simulink model "E33_VCU_simulink"  (R2014a)
settings: Solver=FixedStepDiscrete  StartTime=0.0  StopTime=10.0  FixedStep=0.0005  RelTol=1e-3
values from neighbouring files (symbols this model uses):
  Accu_FAN_Test = ecucoder_cal(Accu_FAN_Test)    [E33_VCU.m]
  Accu_FAN_threshold = ecucoder_cal(Accu_FAN_threshold)    [E33_VCU.m]
  APPS1_Voltage = ecucoder_cal(APPS1_Voltage)    [E33_VCU.m]
  APPS2_Voltage = ecucoder_cal(APPS2_Voltage)    [E33_VCU.m]
  APPS_Map = [0,1000]    [E33_VCU.m]
  APPS_threshold = ecucoder_cal(APPS_threshold)    [E33_VCU.m]
  Beep_Time = ecucoder_cal(Beep_Time)    [E33_VCU.m]
  BeeperTest = ecucoder_cal(BeeperTest)    [E33_VCU.m]
  BMSLedTest = ecucoder_cal(BMSLedTest)    [E33_VCU.m]
  BP_F_threshold = ecucoder_cal(BP_F_threshold)    [E33_VCU.m]
  BP_F_Voltage = ecucoder_cal(BP_F_Voltage)    [E33_VCU.m]
  BP_Map = [0,1000]    [E33_VCU.m]
  BP_R_Voltage = ecucoder_cal(BP_R_Voltage)    [E33_VCU.m]
  Brk_luminance = ecucoder_cal(Brk_luminance)    [E33_VCU.m]
  DCDC_Relay_Test = ecucoder_cal(DCDC_Relay_Test)    [E33_VCU.m]
  FactoryTestEnable = ecucoder_cal(FactoryTestEnable)    [E33_VCU.m]
  HardBrk_luminance = ecucoder_cal(HardBrk_luminance)    [E33_VCU.m]
  IMDLedTest = ecucoder_cal(IMDLedTest)    [E33_VCU.m]
  linear_FL_Map = ecucoder_cal(linear_FL_Map)    [E33_VCU.m]
  linear_FR_Map = ecucoder_cal(linear_FR_Map)    [E33_VCU.m]
  linear_Map = ecucoder_cal(linear_Map)    [E33_VCU.m]
  linear_RL_Map = ecucoder_cal(linear_RL_Map)    [E33_VCU.m]
  linear_RR_Map = ecucoder_cal(linear_RR_Map)    [E33_VCU.m]
  MaxPow = 40    [E33_VCU.m]
  MaxRPM = 5400    [E33_VCU.m]
  MaxRPMchangePerSec = ecucoder_cal(MaxRPMchangePerSec)    [E33_VCU.m]
  MaxTorqChangePerSec = ecucoder_cal(MaxTorqChangePerSec)    [E33_VCU.m]
  Motor_RPM_Map = (0:ceil(MaxRPM/100))*100    [E33_VCU.m]
  Pump_Test = ecucoder_cal(Pump_Test)    [E33_VCU.m]
  Pump_threshold = ecucoder_cal(Pump_threshold)    [E33_VCU.m]
  R2D_Light_Test = ecucoder_cal(R2D_Light_Test)    [E33_VCU.m]
  Radiator_FAN_Test = ecucoder_cal(Radiator_FAN_Test)    [E33_VCU.m]
  SCS_Error_5V = ecucoder_cal(SCS_Error_5V)    [E33_VCU.m]
  SCS_Error_GND = ecucoder_cal(SCS_Error_GND)    [E33_VCU.m]
  SPD_Coef = 1884/40    (= 47.1)    [E33_VCU.m]
  Tail_Light_Test = ecucoder_cal(Tail_Light_Test)    [E33_VCU.m]
  Tmanage_Map = [0,100]    [E33_VCU.m]
  Torq_percentage_Map = Motor_Torq_MAP/MaxTorq*1000    [E33_VCU.m]
libraries: simulink x164, ec55xxlib x44, dspswit3 x6
(part 5 of 5)

== system E33_VCU_simulink/Input/Input/MCU_CAN_Receive/ReceiveMessages/MCU_Stat/MCU_IsFreeMode_Sub ==
  In1 : Inport
  Out1 : Outport
  wires:
  In1/1 -> Out1/1

== system E33_VCU_simulink/Input/Input/MCU_CAN_Receive/ReceiveMessages/MCU_Stat/MCU_IsHvOvervoltage_Sub ==
  In1 : Inport
  Out1 : Outport
  wires:
  In1/1 -> Out1/1

== system E33_VCU_simulink/Input/Input/MCU_CAN_Receive/ReceiveMessages/MCU_Stat/MCU_IsHvUndervoltage_Sub ==
  In1 : Inport
  Out1 : Outport
  wires:
  In1/1 -> Out1/1

== system E33_VCU_simulink/Input/Input/MCU_CAN_Receive/ReceiveMessages/MCU_Stat/MCU_IsLvError_Sub ==
  In1 : Inport
  Out1 : Outport
  wires:
  In1/1 -> Out1/1

== system E33_VCU_simulink/Input/Input/MCU_CAN_Receive/ReceiveMessages/MCU_Stat/MCU_IsMcuNOTActive_Sub ==
  In1 : Inport
  Out1 : Outport
  wires:
  In1/1 -> Out1/1

== system E33_VCU_simulink/Input/Input/MCU_CAN_Receive/ReceiveMessages/MCU_Stat/MCU_IsMcuOvertemp_Sub ==
  In1 : Inport
  Out1 : Outport
  wires:
  In1/1 -> Out1/1

== system E33_VCU_simulink/Input/Input/MCU_CAN_Receive/ReceiveMessages/MCU_Stat/MCU_IsMotorOvertemp_Sub ==
  In1 : Inport
  Out1 : Outport
  wires:
  In1/1 -> Out1/1

== system E33_VCU_simulink/Input/Input/MCU_CAN_Receive/ReceiveMessages/MCU_Stat/MCU_IsOverCurr_Sub ==
  In1 : Inport
  Out1 : Outport
  wires:
  In1/1 -> Out1/1

== system E33_VCU_simulink/Input/Input/MCU_CAN_Receive/ReceiveMessages/MCU_Stat/MCU_IsPreChg_Sub ==
  In1 : Inport
  Out1 : Outport
  wires:
  In1/1 -> Out1/1

== system E33_VCU_simulink/Input/Input/MCU_CAN_Receive/ReceiveMessages/MCU_Stat/MCU_IsReady_Sub ==
  In1 : Inport
  Out1 : Outport
  wires:
  In1/1 -> Out1/1

== system E33_VCU_simulink/Input/Input/MCU_CAN_Receive/ReceiveMessages/MCU_Stat/MCU_IsRevoloverError_Sub ==
  In1 : Inport
  Out1 : Outport
  wires:
  In1/1 -> Out1/1

== system E33_VCU_simulink/Input/Input/MCU_CAN_Receive/ReceiveMessages/MCU_Stat/MCU_IsSelfcheckPass_Sub ==
  In1 : Inport
  Out1 : Outport
  wires:
  In1/1 -> Out1/1

== system E33_VCU_simulink/Input/Input/MCU_CAN_Receive/ReceiveMessages/MCU_Stat/MCU_IsSpdMode_Sub ==
  In1 : Inport
  Out1 : Outport
  wires:
  In1/1 -> Out1/1

== system E33_VCU_simulink/Input/Input/MCU_CAN_Receive/ReceiveMessages/MCU_Stat/MCU_IsTorqMode_Sub ==
  In1 : Inport
  Out1 : Outport
  wires:
  In1/1 -> Out1/1

== system E33_VCU_simulink/Input/Input/MCU_CAN_Receive/ReceiveMessages/MCU_Stat/MCU_IsUnderPowerLim_Sub ==
  In1 : Inport
  Out1 : Outport
  wires:
  In1/1 -> Out1/1

== system E33_VCU_simulink/Input/Input/MCU_CAN_Receive/ReceiveMessages/MCU_Stat/MCU_IsZeroLocMode_Sub ==
  In1 : Inport
  Out1 : Outport
  wires:
  In1/1 -> Out1/1

== system E33_VCU_simulink/Input/Input/MCU_CAN_Receive/ReceiveMessages/MCU_Stat/MCU_SPD_RPT_Sub ==
  In1 : Inport
  Out1 : Outport
  wires:
  In1/1 -> Out1/1

== system E33_VCU_simulink/Input/Input/MCU_CAN_Receive/ReceiveMessages/MCU_Stat/MCU_TORQ_RPT_Sub ==
  In1 : Inport
  Out1 : Outport
  wires:
  In1/1 -> Out1/1

== system E33_VCU_simulink/Input/Input/MCU_CAN_Receive/ReceiveMessages1/Enabled Subsystem/MCU_HvAcCurrRms_Sub ==
  In1 : Inport
  Out1 : Outport
  wires:
  In1/1 -> Out1/1

== system E33_VCU_simulink/Input/Input/MCU_CAN_Receive/ReceiveMessages1/Enabled Subsystem/MCU_HvCurr_Sub ==
  In1 : Inport
  Out1 : Outport
  wires:
  In1/1 -> Out1/1

== system E33_VCU_simulink/Input/Input/MCU_CAN_Receive/ReceiveMessages1/Enabled Subsystem/MCU_HvVolt_Sub ==
  In1 : Inport
  Out1 : Outport
  wires:
  In1/1 -> Out1/1

== system E33_VCU_simulink/Input/Input/MCU_CAN_Receive/ReceiveMessages1/Enabled Subsystem/MCU_McuTemp_Sub ==
  In1 : Inport
  Out1 : Outport
  wires:
  In1/1 -> Out1/1

== system E33_VCU_simulink/Input/Input/MCU_CAN_Receive/ReceiveMessages1/Enabled Subsystem/MCU_MotorTemp_Sub ==
  In1 : Inport
  Out1 : Outport
  wires:
  In1/1 -> Out1/1

== stateflow chart E33_VCU_simulink/Subsystem1/TmanageCtrl/Accu_FAN1 ==
  state LEDStat
    state Run
      du:FanDutyCycl = FanPwr
    state Init
    state PumpTest
      du:FanDutyCycl  = uint16(GetDutyCyc(temporalCount(sec),8));
    (default) -> Init
    Init -> PumpTest : after(1,sec)
    Run -> PumpTest : [IsPrechg]
    PumpTest -> Run : [after(2,sec)]
  data: elapsed_sec function_input; DutyCyc function_output uint8; period function_input; FanPwr input uint16; FanDutyCycl output uint16; IsPrechg input boolean; IsRun input
  function DutyCyc = GetDutyCyc(elapsed_sec, period):
    | function DutyCyc = GetDutyCyc(elapsed_sec, period)
    |     DutyCyc = 25.*sin(2.*pi.*(elapsed_sec./period+0.75))+25;      %Note: sin in rad
    | end

== stateflow chart E33_VCU_simulink/Function-Call Subsystem/R2D_State/Chart ==
  state VehStat [parallel]
    settings: executionOrder=1
    state Guard
    state Standby
    state WaitForEngine
    state Trans
    state Init
    state Ready
    Standby -> Guard [order 1] : [R2D_SW&&BP_F_OK&&APPS_OK]
    Guard -> Trans [order 1] : after(0.25,sec){send(EbeepON,BeeperStat)}
    WaitForEngine -> Standby : [MCU_Ready]
    Standby -> WaitForEngine [order 2] : [~MCU_Ready]
    Guard -> Standby [order 2] : [~R2D_SW||~BP_F_OK||~APPS_OK]
    Init -> WaitForEngine : [after(1,sec)]
    Ready -> WaitForEngine : [~MCU_Ready]
    Guard -> WaitForEngine [order 3] : [~MCU_Ready]
    Trans -> Ready : after(Beep_Time,sec){send(EbeepOFF,BeeperStat)}
    (default) -> Init
  state Output [parallel]
    du:
    VehStandby = in(VehStat.Standby);
    VehReady = in(VehStat.Ready);
    BeeperStOut = in(BeeperStat.ON);
    settings: executionOrder=3
  state BeeperStat [parallel]
    settings: executionOrder=2
    state OFF
    state ON
    (default) -> OFF
    OFF -> ON : EbeepON
    ON -> OFF : EbeepOFF
  data: BeeperStOut output boolean size=1; VehStandby output boolean; R2D_SW input boolean; APPS_OK input boolean; BP_F_OK input boolean; MCU_Ready input boolean; VehReady output boolean; Beep_Time input
  events: EbeepON local FUNCTION_CALL_EVENT; EbeepOFF local FUNCTION_CALL_EVENT

== stateflow chart E33_VCU_simulink/Subsystem1/TailLight/LED ==
  state LEDStat
    state Init
    state LightTest
      du:LEDDutyCyc  = uint16(GetDutyCyc(temporalCount(sec),4));
    state OFF
      entry: LEDDutyCyc = uint16(0);
    state Blink
      state BlinkOn
        entry: LEDDutyCyc = uint16(HardBrk_luminance);
      state BlinkOff
        entry: LEDDutyCyc = uint16(Brk_luminance);
      (default) -> BlinkOn
      BlinkOn -> BlinkOff : after(100,msec)
      BlinkOff -> BlinkOn : after(100,msec)
    state ON
      entry: LEDDutyCyc = uint16(Brk_luminance);
    (default) -> Init
    Init -> LightTest : after(1,sec)
    LightTest -> OFF : after(4,sec){LEDDutyCyc = uint16(0)}
    OFF -> Blink [order 1] : [IsHardBrk]
    Blink -> OFF [order 2] : [~IsBrk]
    OFF -> ON [order 2] : [IsBrk]
    ON -> OFF [order 1] : [~IsBrk]
    Blink -> ON [order 1] : [~IsHardBrk&&IsBrk]
    ON -> Blink [order 2] : [IsHardBrk]
  data: elapsed_sec function_input; DutyCyc function_output uint8; period function_input; IsBrk input boolean; LEDDutyCyc output uint16; IsHardBrk input boolean; Brk_luminance input double; HardBrk_luminance input double
  function DutyCyc = GetDutyCyc(elapsed_sec, period):
    | function DutyCyc = GetDutyCyc(elapsed_sec, period)
    |     DutyCyc = 25.*sin(2.*pi.*(elapsed_sec./period+0.75))+25;      %Note: sin in rad
    | end

== stateflow chart E33_VCU_simulink/Subsystem1/TmanageCtrl/Pump ==
  state Pump_MR
    state Init
    state OFF
      du:Pump_ON = 0
    state ON
      du:Pump_ON = 1
    state PumpTest
      du:Pump_ON  =  1
    (default) -> Init
    Init -> PumpTest : after(1,sec)
    OFF -> ON : [Pump_OK]
    PumpTest -> OFF : after(8,sec)
    ON -> OFF : [~Pump_OK]
  data: Pump_OK input boolean; MCU_IsReady input boolean; Pump_ON output

== stateflow chart E33_VCU_simulink/Subsystem1/PanelCtrl/Ready_SW ==
  state LEDStat
    state Blink
      state BlinkONslow
        entry: R2D_Light = true;
      state BlinkOFFslow
        entry: R2D_Light = false;
      (default) -> BlinkONslow
      BlinkONslow -> BlinkOFFslow : [after(1,sec)]
      BlinkOFFslow -> BlinkONslow : [after(1,sec)]
    state Init
      du: R2D_Light = false;
    state Test
      en:
      R2D_Light = true;
    state FastBlink
      state BlinkONfast
        entry: R2D_Light = true;
      state BlinkOFFfast
        entry: R2D_Light = false;
      (default) -> BlinkONfast
      BlinkONfast -> BlinkOFFfast : after(0.2,sec)
      BlinkOFFfast -> BlinkONfast : after(0.2,sec)
    state ON
      en:R2D_Light = true;
    state OFF
      en:R2D_Light = false;
    (junction 72) -> (junction 51)
    (junction 51) -> (junction 70)
    (junction 82) -> (junction 72)
    (default) -> Init
    Init -> Test : after(1,sec)
    Test -> (junction 70) : after(3,sec){R2D_Light = false}
    (junction 70) -> Blink [order 1] : [VehStandby]
    Blink -> (junction 82) : [APPS_Unreliable||~VehStandby]
    (junction 70) -> (junction 93) [order 2]
    (junction 96) -> (junction 82)
    (junction 93) -> FastBlink [order 1] : [APPS_Unreliable]
    FastBlink -> (junction 96) : [~APPS_Unreliable]
    (junction 78) -> (junction 96)
    (junction 93) -> (junction 73) [order 2]
    (junction 73) -> ON [order 1] : [VehReady]
    ON -> (junction 78)
    (junction 73) -> (junction 67) [order 2]
    (junction 59) -> (junction 78)
    (junction 67) -> OFF
    OFF -> (junction 59)
  data: R2D_Light output boolean; APPS_Unreliable input boolean; VehStandby input boolean; VehReady input boolean

== stateflow chart E33_VCU_simulink/Subsystem1/PanelCtrl/BMS_ALM ==
  state LEDStat
    state AlevelAlm
      en:LED = true;
    state Init
      en:
      LED = false;
    state BlevelAlm
      state BlvBlinkOff
        entry:
        LED = false;
      state BlvBlinkON
        entry:
        LED = true;
      BlvBlinkOff -> BlvBlinkON : after(1,sec)
      BlvBlinkON -> BlvBlinkOff : after(1,sec)
      (default) -> BlvBlinkON
    state Test
      en:
      LED = true;
    state OFF
      en:
      LED = false;
    (junction 55) -> (junction 56)
    (junction 56) -> (junction 15)
    (junction 47) -> (junction 55)
    (default) -> Init
    Test -> (junction 15) : after(3,sec){LED = true}
    (junction 15) -> AlevelAlm [order 1] : [AlmLv==1||~OK]
    (junction 15) -> (junction 32) [order 2]
    AlevelAlm -> (junction 47) : [AlmLv~=1&&OK]
    (junction 45) -> (junction 47)
    Init -> Test : after(1,sec)
    (junction 32) -> BlevelAlm [order 1] : [AlmLv==2]
    (junction 32) -> (junction 34) [order 2]
    BlevelAlm -> (junction 45) : [AlmLv~=2||~OK]
    (junction 41) -> (junction 45)
    (junction 34) -> OFF
    OFF -> (junction 41)
  data: AlmLv input; LED output boolean; OK input

== stateflow chart E33_VCU_simulink/Subsystem1/PanelCtrl/IMD_ALM ==
  state LEDStat
    state AlevelAlm
      en:LED = false;
    state Init
      en:
      LED = false;
    state OFF
      en:
      LED = true;
    state Test
      en:
      LED = true;
    (junction 55) -> (junction 56)
    (junction 56) -> (junction 15)
    (junction 47) -> (junction 55)
    (default) -> Init
    (junction 15) -> AlevelAlm [order 1] : [~OK]
    Test -> (junction 15) : after(3,sec){LED = true}
    (junction 15) -> (junction 34) [order 2]
    AlevelAlm -> (junction 47) : [OK]
    (junction 41) -> (junction 47)
    Init -> Test : after(1,sec)
    (junction 34) -> OFF
    OFF -> (junction 41)
  data: LED output boolean; OK input

== stateflow chart E33_VCU_simulink/Subsystem1/DCDC_Ctrl/DCDC_Ctrl ==
  state DCDC_MR
    du:DCDC_ON = in(DCDC_MR.ON)
    state OFF
    state ON
    (default) -> OFF
    OFF -> ON : [after(2,sec)&&HV_ON]
    ON -> OFF : [after(2,sec)&&~HV_ON]
  data: HV_ON input boolean; DCDC_ON output boolean

== stateflow chart E33_VCU_simulink/Subsystem1/TmanageCtrl/Accu_FAN ==
  state LEDStat
    state Run
      du:FanDutyCycl = FanPwr
    state Init
    state Ready_to_close
      du:FanDutyCycl = FanPwr
    state PumpTest
      du:FanDutyCycl  = uint16(GetDutyCyc(temporalCount(sec),8));
    state Stand
      du: FanDutyCycl = uint16(0);
    (default) -> Init
    Stand -> Run : [IsRun||after(3,sec)]
    Run -> Ready_to_close : [~IsRun]
    Init -> PumpTest : after(1,sec)
    Ready_to_close -> Stand : [after(30,sec)||IsPrechg]
    PumpTest -> Stand : {FanDutyCycl = uint16(0)}
  data: elapsed_sec function_input; DutyCyc function_output uint8; period function_input; FanPwr input uint16; FanDutyCycl output uint16; IsPrechg input boolean; IsRun input
  function DutyCyc = GetDutyCyc(elapsed_sec, period):
    | function DutyCyc = GetDutyCyc(elapsed_sec, period)
    |     DutyCyc = 25.*sin(2.*pi.*(elapsed_sec./period+0.75))+25;      %Note: sin in rad
    | end
